simulink model "gradient_model"  (R2025a)
settings: Solver=VariableStepAuto  StartTime=0.0  StopTime=50  RelTol=1e-3
values from neighbouring files (symbols this model uses):
  Tf = 1    [gradient.m]    (also in mse.m)
settings Model: Creator=Korisnik  LastModifiedBy=Korisnik

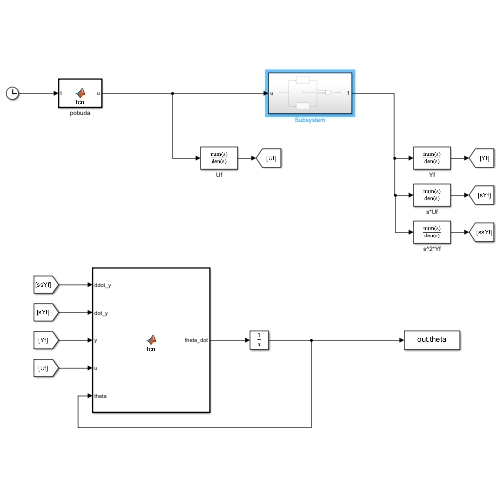
[thumbnail: Simulink's stored preview of the top-level diagram]
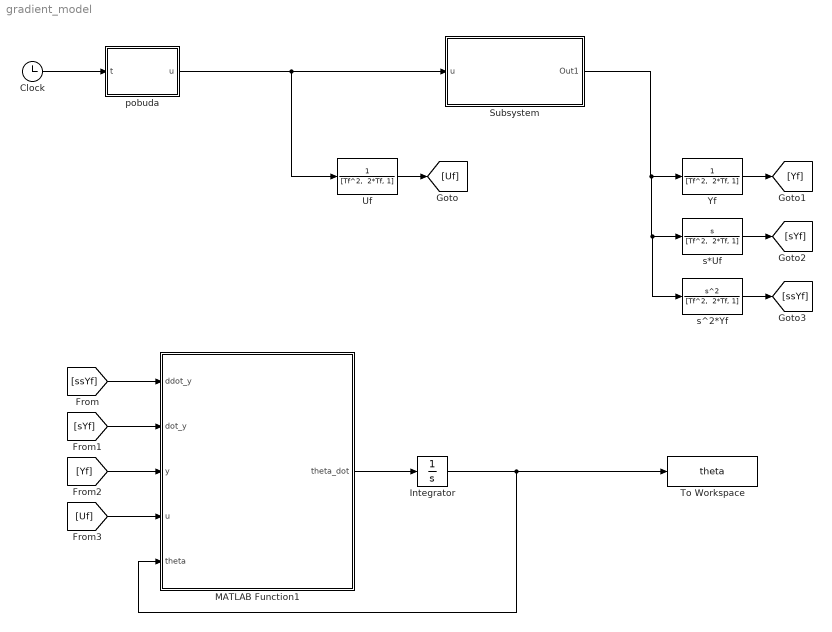
== system gradient_model ==
  Clock : Clock
  Integrator : Integrator  InitialCondition=[0; 0; 0]
  MATLAB Function1 : MATLAB Function  TreatAsAtomicUnit=on
  Subsystem : Subsystem
  To Workspace : ToWorkspace  VariableName=theta  SaveFormat=Timeseries  SampleTime=-1
  Uf : TransferFcn  Denominator="[Tf^2,  2*Tf, 1]"
  Yf : TransferFcn  Denominator="[Tf^2,  2*Tf, 1]"
  pobuda : MATLAB Function  TreatAsAtomicUnit=on
  s*Uf : TransferFcn  Numerator=[1, 0]  Denominator="[Tf^2,  2*Tf, 1]"
  s^2*Yf : TransferFcn  Numerator=[1, 0, 0]  Denominator="[Tf^2,  2*Tf, 1]"
  wires:
  s^2*Yf/1 -> [ssYf]
  Uf/1 -> [Uf]
  MATLAB Function1/1(theta_dot) -> Integrator/1
  Yf/1 -> [Yf]
  pobuda/1(u) -> Subsystem/1(u), Uf/1
  [ssYf] -> MATLAB Function1/1(ddot_y)
  s*Uf/1 -> [sYf]
  [Yf] -> MATLAB Function1/3(y)
  [sYf] -> MATLAB Function1/2(dot_y)
  Integrator/1 -> To Workspace/1, MATLAB Function1/5(theta)
  [Uf] -> MATLAB Function1/4(u)
  Subsystem/1(Out1) -> s^2*Yf/1, s*Uf/1, Yf/1
  Clock/1 -> pobuda/1(t)

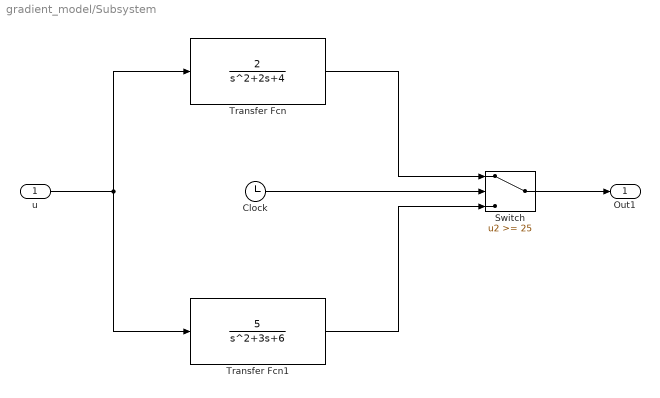
== system gradient_model/Subsystem ==
  u : Inport
  Clock : Clock
      settings: Decimation=5
  Switch : Switch  Threshold=25  SaturateOnIntegerOverflow=off  InputSameDT=off
  Transfer Fcn : TransferFcn  Numerator=2  Denominator=[1,2, 4]
  Transfer Fcn1 : TransferFcn  Numerator=5  Denominator=[1, 3, 6]
  Out1 : Outport
  wires:
  Clock/1 -> Switch/2
  u/1 -> Transfer Fcn1/1, Transfer Fcn/1
  Transfer Fcn/1 -> Switch/1
  Transfer Fcn1/1 -> Switch/3
  Switch/1 -> Out1/1

== matlab function gradient_model/MATLAB Function1 ==
  data: ddot_y input; dot_y input; y input; u input; theta_dot output; theta input
% kod sa casa
function theta_dot = fcn(ddot_y, dot_y, y, u, theta)
    p = [-dot_y; -y; u];
    eta = ddot_y;

    G = 12000 * eye(length(p), length(p));

    theta_dot = G * p * (eta - p' * theta);
end

== matlab function gradient_model/pobuda ==
  data: t input; u output
function u = fcn(t)
    u = 0;
    fmax = 5;
    for i = 1:fmax
        u = u + sin(2 * pi * i * t);
    end
